simulink model "Robotk_FSM_"  (R2020b)
settings: Solver=FixedStepDiscrete  StartTime=0.0  StopTime=8  FixedStep=0.1  RelTol=1e-3  EnableMultiTasking=on
settings Model: EnablePacing=on  Creator=HP  LastModifiedBy=HP
settings SolverCC: AutoInsertRateTranBlk=on
settings DataIOCC: LimitDataPoints=on
settings OptimizationCC: LifeSpan=inf
settings DebuggingCC: AllowSymbolicDim=off  SFUnexpectedBacktrackingDiag=warning  SFNoUnconditionalDefaultTransitionDiag=warning  SFExecutionAtInitializationDiag=none  SFMachineParentedDataDiag=error  ArithmeticOperatorsInVariantConditions=warning
settings SFSimCC: SimUseLocalCustomCode=off  CustomCodeUndefinedFunction=UseInterfaceOnly
settings RTWCC: RTWUseLocalCustomCode=off
settings CodeAppCC: StateflowObjectComments=on
settings GRTTargetCC: TargetLangStandard=C89/C90 (ANSI)
settings ConfigComp: CovMetricSettings=dw  CovSaveCumulativeToWorkspaceVar=on  CovSaveSingleToWorkspaceVar=on  CovExternalEMLEnable=off  CovSFcnEnable=off

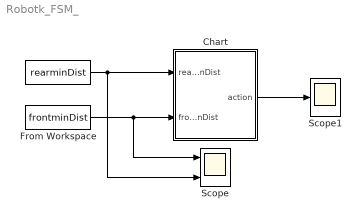
== system Robotk_FSM_ ==
  " " : FromWorkspace  VariableName=rearminDist  SampleTime=-1
  Chart : Stateflow chart  TreatAsAtomicUnit=on
  From Workspace : FromWorkspace  VariableName=frontminDist  SampleTime=-1
  Scope : Scope  NumInputPorts=2
  Scope1 : Scope
  wires:
  From Workspace/1 -> Scope/1, Chart/2(frontminDist)
  " "/1 -> Scope/2, Chart/1(rearminDist)
  Chart/1(action) -> Scope1/1

== stateflow chart Robotk_FSM_/Chart ==
  state EMERGENCY_STOP
    entry:
    emergencyTime=0;
    action = FSMStates.EMERGENCY_STOP;
    during:
    emergencyTime = emergencyTime + 1;
  state FORWARD
    entry :
    last_state = FSMStates.FORWARD;
    action = FSMStates.FORWARD;
  state REVERSE_AND_CHECK
    entry :
    last_state = FSMStates.REVERSE_AND_CHECK;
    action = FSMStates.REVERSE_AND_CHECK;
    reverse_time = 0;
    during :
    reverse_time = reverse_time + 1;
  state SLOWING_DOWN
    entry :
    last_state = FSMStates.SLOWING_DOWN;
    action = FSMStates.SLOWING_DOWN;
    slow_time = 0;
    during :
    slow_time = slow_time + 1;
  state STOP
    entry :
    action = FSMStates.STOP;
    stopTime = 0;
    during:
    stopTime = stopTime + 1;
  state TURNING
    entry :
    last_state = FSMStates.TURNING;
    action = FSMStates.TURNING;
    turningTime = 0;
    during :
    turningTime = turningTime + 1;
  REVERSE_AND_CHECK -> EMERGENCY_STOP [order 1] : [rearminDist <= CRITICAL_DIST ]
  FORWARD -> EMERGENCY_STOP [order 1] : [frontminDist <= CRITICAL_DIST]
  EMERGENCY_STOP -> STOP [order 1] : [frontminDist <= CRITICAL_DIST && rearminDist <= CRITICAL_DIST && emergencyTime == EMERGENCY_DURATION]
  TURNING -> EMERGENCY_STOP [order 1] : [frontminDist <= CRITICAL_DIST]
  SLOWING_DOWN -> EMERGENCY_STOP [order 2] : [frontminDist <= CRITICAL_DIST]
  EMERGENCY_STOP -> (junction 70) [order 2] : [frontminDist > 3 &&  emergencyTime >= EMERGENCY_DURATION]
  (default) -> FORWARD
  (junction 70) -> FORWARD [order 2] : [last_state == FSMStates.FORWARD]
  (junction 70) -> REVERSE_AND_CHECK [order 3] : [rearminDist > CRITICAL_DIST  && last_state == FSMStates.REVERSE_AND_CHECK]
  (junction 70) -> TURNING [order 4] : [last_state == FSMStates.TURNING]
  (junction 70) -> SLOWING_DOWN [order 1] : [last_state == FSMStates.SLOWING_DOWN]
  REVERSE_AND_CHECK -> STOP [order 2] : [frontminDist <=CRITICAL_DIST && rearminDist <=CRITICAL_DIST]
  STOP -> FORWARD [order 2] : [frontminDist > ACCEPTABLE_DIST]
  SLOWING_DOWN -> FORWARD [order 3] : [frontminDist > ACCEPTABLE_DIST]
  SLOWING_DOWN -> STOP [order 1] : [frontminDist <= ACCEPTABLE_DIST && frontminDist > CRITICAL_DIST && slow_time >= slow_duration]
  STOP -> REVERSE_AND_CHECK [order 1] : [frontminDist <= ACCEPTABLE_DIST && stopTime >= STOP_DURATION]
  FORWARD -> SLOWING_DOWN [order 2] : [frontminDist <= ACCEPTABLE_DIST && frontminDist > CRITICAL_DIST]
  TURNING -> STOP [order 3] : [turningTime >= TURNING_DURATION]
  TURNING -> FORWARD [order 2] : [frontminDist >=SAFE_DIST && turningTime >= TURNING_DURATION ]
  REVERSE_AND_CHECK -> TURNING [order 3] : [rearminDist >= SAFE_DIST && reverse_time >= reverse_duration]
  data: last_state local Enum: FSMStates; rearminDist input; emergencyTime local; stopTime local; turningTime local; action output Enum: FSMStates; CRITICAL_DIST constant double =3; SAFE_DIST constant double =15; TURNING_DURATION constant double =2; EMERGENCY_DURATION constant double =2; STOP_DURATION constant double =2; reverse_time local; reverse_duration constant double; frontminDist input; slow_time local; slow_duration constant double =2; ACCEPTABLE_DIST constant double =8
